simulink model "MLP_networks"  (Simulink 7.7)
settings: Solver=ode45  StartTime=0.0  StopTime=10.0  RelTol=1e-3
libraries: neural x1629
(part 25 of 39)

== system MLP_networks/net_col_e_f_4_5/Layer 2/LW{2,1} ==
  "ad{2,1}" : Inport  PortDimensions=20
      mask Display: e = 0.06;c1 = [120 230 180]/255;c2 = ([120 230 180]+0)/(256+128);c3 = ([120 230 180]+128)/(256+128);patch([0 1 1 0],[0 0 1 1],c1);patch([0 1 1 1-e 1-e 0+e],[0 0 1 1-e 0+e 0+e],c2);patch([0 0 1 1-e 0+e 0+e],[0 1 1 1-e 1-e 0+e],c3);plot([0 1 1 0 0],[0 0 1 1 0]);
  "IW{2,1}(1,:)'" : Constant  Value=[-0.45151548886161508;0.25536682711089687;-0.34681685037556653;-0.34392706874455214;-0.027803182510490278;0.41746512687912851;0.55437397851143355;0.083610404804986299;-0.25747534404557321;-0.31935504733540621;-0.59689163525306344;-0.045683988316651554;-0.43964163854361554;0.11284189827815641;-0.64222573757867818;-0.35635141759648353;0.12263688035408589;-0.58273881801377925;-0.46555293587298402;-0.0080108450108429229]
      mask Display: e = 0.06;c1 = [120 150 230]/255;c2 = ([120 150 230]+0)/383;c3 = ([120 150 230]+128)/383;patch([0 1 1 0],[0 0 1 1],c1);patch([0 1 1 1-e 1-e 0+e],[0 0 1 1-e 0+e 0+e],c2);patch([0 0 1 1-e 0+e 0+e],[0 1 1 1-e 1-e 0+e],c3);plot([0 1 1 0 0],[0 0 1 1 0]);disp('weights');
  "IW{2,1}(10,:)'" : Constant  Value=[0.41523421292602436;-0.079325917445633137;0.60054028682480187;0.54825507956649056;0.042245915117327067;-0.22239028106970385;-0.15170393677920968;-0.28769964161831629;-0.66009683615917791;0.48814562672504147;0.04655942021694514;0.68149765275244589;-0.062084447563797093;-0.47323297326885766;0.22267393118045514;-0.3678342526120863;-0.22194063098682851;0.37035750995645711;0.12347763221984454;-0.31522257591675068]
      mask Display: e = 0.06;c1 = [120 150 230]/255;c2 = ([120 150 230]+0)/383;c3 = ([120 150 230]+128)/383;patch([0 1 1 0],[0 0 1 1],c1);patch([0 1 1 1-e 1-e 0+e],[0 0 1 1-e 0+e 0+e],c2);patch([0 0 1 1-e 0+e 0+e],[0 1 1 1-e 1-e 0+e],c3);plot([0 1 1 0 0],[0 0 1 1 0]);disp('weights');
  "IW{2,1}(11,:)'" : Constant  Value=[0.22051107884975904;0.04667985599907265;-0.42900276186151998;-0.61671126003943155;-0.42621721318611683;-0.18489691728747051;-0.13777397473069228;-0.037474895097715587;0.51799599312536593;-0.084083188529973152;-0.64644464204408958;-0.01135044235336753;-0.070911414979821383;-0.17601825270858257;0.61930700333124977;-0.082126080553112879;0.63071072678260498;0.16527980798998046;0.56344172772425338;0.37422462011786845]
      mask Display: e = 0.06;c1 = [120 150 230]/255;c2 = ([120 150 230]+0)/383;c3 = ([120 150 230]+128)/383;patch([0 1 1 0],[0 0 1 1],c1);patch([0 1 1 1-e 1-e 0+e],[0 0 1 1-e 0+e 0+e],c2);patch([0 0 1 1-e 0+e 0+e],[0 1 1 1-e 1-e 0+e],c3);plot([0 1 1 0 0],[0 0 1 1 0]);disp('weights');
  "IW{2,1}(12,:)'" : Constant  Value=[-0.084493713905112233;0.48678115841687936;0.45142563808834973;-0.36811298581343271;-0.40924916828354552;0.17807058636038001;-0.46456329081936826;0.42281416037711955;0.20377516377164831;0.47843783198352607;-0.26407473415439514;-0.10465597364986522;-0.47919068721275565;0.31496744878274513;0.20713329388106066;0.49180314424343141;0.57605572335121114;-0.22625235422828688;0.46448345523528134;0.27110377760943549]
      mask Display: e = 0.06;c1 = [120 150 230]/255;c2 = ([120 150 230]+0)/383;c3 = ([120 150 230]+128)/383;patch([0 1 1 0],[0 0 1 1],c1);patch([0 1 1 1-e 1-e 0+e],[0 0 1 1-e 0+e 0+e],c2);patch([0 0 1 1-e 0+e 0+e],[0 1 1 1-e 1-e 0+e],c3);plot([0 1 1 0 0],[0 0 1 1 0]);disp('weights');
  "IW{2,1}(13,:)'" : Constant  Value=[-0.30149359766207418;-0.45992478689272992;0.37870307637329009;0.33785088301701416;0.29211040783918429;0.418882893877153;0.52364539021317746;0.22698130724798568;0.41621078446985132;0.32359159164504292;-0.37444769328437505;-0.41424018215945352;0.45640798227554841;0.47255964818598079;0.063960542335897014;-0.33017321165220542;0.25384780898493198;-0.47685133154288806;0.15216466743509105;-0.52149157749906128]
      mask Display: e = 0.06;c1 = [120 150 230]/255;c2 = ([120 150 230]+0)/383;c3 = ([120 150 230]+128)/383;patch([0 1 1 0],[0 0 1 1],c1);patch([0 1 1 1-e 1-e 0+e],[0 0 1 1-e 0+e 0+e],c2);patch([0 0 1 1-e 0+e 0+e],[0 1 1 1-e 1-e 0+e],c3);plot([0 1 1 0 0],[0 0 1 1 0]);disp('weights');
  "IW{2,1}(14,:)'" : Constant  Value=[-0.28930249915012268;-0.44091010774765055;0.27168073044539698;0.49942675426286448;0.20512264087672194;-0.37602605346876733;-0.13189155517247578;-0.23130337724636571;0.094450964076811791;-0.16998091204382224;0.16016055355889927;-0.60759126781458894;0.43104902085232288;-0.56965892606835733;0.17809072069355344;0.28659787509126711;-0.4614072071044088;0.34603812505852033;0.46450688890271252;0.62315023418671689]
      mask Display: e = 0.06;c1 = [120 150 230]/255;c2 = ([120 150 230]+0)/383;c3 = ([120 150 230]+128)/383;patch([0 1 1 0],[0 0 1 1],c1);patch([0 1 1 1-e 1-e 0+e],[0 0 1 1-e 0+e 0+e],c2);patch([0 0 1 1-e 0+e 0+e],[0 1 1 1-e 1-e 0+e],c3);plot([0 1 1 0 0],[0 0 1 1 0]);disp('weights');
  "IW{2,1}(15,:)'" : Constant  Value=[0.15751683268771688;0.4192261852453415;-0.016011679153426196;0.41859753641114317;0.25793731142113935;0.18105600414691669;-0.053963693799016686;-0.56399142195908658;0.28049437874349148;-0.35138609966460516;0.27311840894612877;-0.17274187268768235;-0.23510480251311197;0.61360552858247386;0.73129244534754589;-0.70291713895824193;0.46749838984635617;-0.20341619662205515;0.021850222878550853;-0.12862670708565105]
      mask Display: e = 0.06;c1 = [120 150 230]/255;c2 = ([120 150 230]+0)/383;c3 = ([120 150 230]+128)/383;patch([0 1 1 0],[0 0 1 1],c1);patch([0 1 1 1-e 1-e 0+e],[0 0 1 1-e 0+e 0+e],c2);patch([0 0 1 1-e 0+e 0+e],[0 1 1 1-e 1-e 0+e],c3);plot([0 1 1 0 0],[0 0 1 1 0]);disp('weights');
  "IW{2,1}(16,:)'" : Constant  Value=[-0.27657012366938966;0.15371322358443629;-0.55363356208853609;0.36378906637276537;0.52464494926328686;0.28784110928429885;0.46469559105081931;0.15025065447007821;-0.33039322751314137;-0.06464765041817773;0.20119553589259553;0.133449729104959;0.45132776068432545;0.34991929216206841;-0.40133073823107779;-0.39379744327608268;0.53901406218322345;-0.45996647999988743;-0.4115733283149775;-0.50627799265694229]
      mask Display: e = 0.06;c1 = [120 150 230]/255;c2 = ([120 150 230]+0)/383;c3 = ([120 150 230]+128)/383;patch([0 1 1 0],[0 0 1 1],c1);patch([0 1 1 1-e 1-e 0+e],[0 0 1 1-e 0+e 0+e],c2);patch([0 0 1 1-e 0+e 0+e],[0 1 1 1-e 1-e 0+e],c3);plot([0 1 1 0 0],[0 0 1 1 0]);disp('weights');
  "IW{2,1}(17,:)'" : Constant  Value=[-0.29644152955930081;-0.4308597944950418;-0.54634565930104229;0.58330284826123979;-0.10928909899825232;0.56925501441853865;0.57554506008322792;0.53497171762174578;0.55505559616470479;-0.1148742286263794;-0.53564900218664824;0.044535446781484522;0.20798460923717371;0.29893088797223188;-0.21469482723072089;0.19037112584674373;-0.11652538868178051;0.13763581536126696;0.31150300464310915;-0.094213883008351984]
      mask Display: e = 0.06;c1 = [120 150 230]/255;c2 = ([120 150 230]+0)/383;c3 = ([120 150 230]+128)/383;patch([0 1 1 0],[0 0 1 1],c1);patch([0 1 1 1-e 1-e 0+e],[0 0 1 1-e 0+e 0+e],c2);patch([0 0 1 1-e 0+e 0+e],[0 1 1 1-e 1-e 0+e],c3);plot([0 1 1 0 0],[0 0 1 1 0]);disp('weights');
  "IW{2,1}(18,:)'" : Constant  Value=[0.35417996583849992;0.15868067448218406;-0.35585371797525295;-0.21707074271476465;-0.30874927399822116;0.28469132401145908;0.35472209819061928;0.3415908850634099;-0.55469444381337141;0.35094451772152646;0.70640754781705073;-0.75008386250934855;-0.4794943931696436;-0.21128936679171628;-0.12072435755185078;0.12920961420023977;-0.49022617267297025;-0.38439863878407654;0.21885884977322467;-0.16430755827177285]
      mask Display: e = 0.06;c1 = [120 150 230]/255;c2 = ([120 150 230]+0)/383;c3 = ([120 150 230]+128)/383;patch([0 1 1 0],[0 0 1 1],c1);patch([0 1 1 1-e 1-e 0+e],[0 0 1 1-e 0+e 0+e],c2);patch([0 0 1 1-e 0+e 0+e],[0 1 1 1-e 1-e 0+e],c3);plot([0 1 1 0 0],[0 0 1 1 0]);disp('weights');
  "IW{2,1}(19,:)'" : Constant  Value=[-0.27337498067941102;-0.56335228384022429;-0.053155904668951752;-0.34417360501701988;-0.43978832790699596;-0.5760611884699075;-0.022993975155131994;0.51733797376312773;-0.59073422965442535;-0.32599506194253752;0.39691334336237133;0.59730593053673864;0.51579578103074142;0.18622803089423495;0.22952335035122878;0.28644120269709844;-0.022213765514939521;0.70000625526608418;-0.18510048875217902;0.13283311097415057]
      mask Display: e = 0.06;c1 = [120 150 230]/255;c2 = ([120 150 230]+0)/383;c3 = ([120 150 230]+128)/383;patch([0 1 1 0],[0 0 1 1],c1);patch([0 1 1 1-e 1-e 0+e],[0 0 1 1-e 0+e 0+e],c2);patch([0 0 1 1-e 0+e 0+e],[0 1 1 1-e 1-e 0+e],c3);plot([0 1 1 0 0],[0 0 1 1 0]);disp('weights');
  "IW{2,1}(2,:)'" : Constant  Value=[0.28437748977449745;0.25833400523463534;-0.037021315231732362;-0.68497084905838668;0.41852802820217722;-0.57834088769097802;0.56203903722750315;-0.21187070828271204;-0.10478414525478082;0.57659603478192067;-0.7418424500897558;-0.39611970693280452;0.069829662330228442;-0.15617944332060318;0.25357993180904392;-0.065271231016431744;0.31908541214869918;-0.060339638688504026;0.081335933949920322;-0.37526662583148929]
      mask Display: e = 0.06;c1 = [120 150 230]/255;c2 = ([120 150 230]+0)/383;c3 = ([120 150 230]+128)/383;patch([0 1 1 0],[0 0 1 1],c1);patch([0 1 1 1-e 1-e 0+e],[0 0 1 1-e 0+e 0+e],c2);patch([0 0 1 1-e 0+e 0+e],[0 1 1 1-e 1-e 0+e],c3);plot([0 1 1 0 0],[0 0 1 1 0]);disp('weights');
  "IW{2,1}(20,:)'" : Constant  Value=[-0.64409750347750527;0.34646163018063469;-0.58798361872778426;0.0085129432317137699;-0.45090915364862233;-0.30265599114041347;0.0077096397280898114;0.26412412391892426;0.086341121032416118;-0.30548428858564097;0.3660050363044266;-0.62694176855105233;-0.48252047203090886;-0.52245941640535487;0.38730598212166212;-0.064531981023332644;0.17425424198955766;0.53562209298160957;-0.061191832450063051;0.043829994940977078]
      mask Display: e = 0.06;c1 = [120 150 230]/255;c2 = ([120 150 230]+0)/383;c3 = ([120 150 230]+128)/383;patch([0 1 1 0],[0 0 1 1],c1);patch([0 1 1 1-e 1-e 0+e],[0 0 1 1-e 0+e 0+e],c2);patch([0 0 1 1-e 0+e 0+e],[0 1 1 1-e 1-e 0+e],c3);plot([0 1 1 0 0],[0 0 1 1 0]);disp('weights');
  "IW{2,1}(21,:)'" : Constant  Value=[-0.080332203363595853;0.37070858702897092;0.23410866955263651;0.26082762551266808;-0.46717907369368694;-0.50512936006521436;0.45092995928204604;-0.51896037678346807;-0.56100829375195771;0.21814326179802759;0.040103435817852924;0.17387153933872629;-0.13079318849718519;0.61280554963107803;-0.31277142209582232;-0.39206937616288345;0.37537171334969721;-0.075970000529032425;0.41224430106766913;0.52254642336293189]
      mask Display: e = 0.06;c1 = [120 150 230]/255;c2 = ([120 150 230]+0)/383;c3 = ([120 150 230]+128)/383;patch([0 1 1 0],[0 0 1 1],c1);patch([0 1 1 1-e 1-e 0+e],[0 0 1 1-e 0+e 0+e],c2);patch([0 0 1 1-e 0+e 0+e],[0 1 1 1-e 1-e 0+e],c3);plot([0 1 1 0 0],[0 0 1 1 0]);disp('weights');
  "IW{2,1}(22,:)'" : Constant  Value=[-0.42704336720470931;-0.30041882948731219;0.3956809292562421;-0.16971732971577322;0.076497757409530881;-0.47929628792147649;-0.24193017744364609;-0.247136213895218;0.07517234050153429;0.10672754370040455;-0.36319238605476445;0.97284045806936903;0.048026106182699771;0.42305021233232182;-0.46384915148240169;-0.41910492272950939;-0.64315109777288715;-0.4816034710376344;-0.1382623929613658;0.43671260004494816]
      mask Display: e = 0.06;c1 = [120 150 230]/255;c2 = ([120 150 230]+0)/383;c3 = ([120 150 230]+128)/383;patch([0 1 1 0],[0 0 1 1],c1);patch([0 1 1 1-e 1-e 0+e],[0 0 1 1-e 0+e 0+e],c2);patch([0 0 1 1-e 0+e 0+e],[0 1 1 1-e 1-e 0+e],c3);plot([0 1 1 0 0],[0 0 1 1 0]);disp('weights');
  "IW{2,1}(23,:)'" : Constant  Value=[0.43259582298602201;0.085300864815750416;-0.066611187728102428;-0.46644934301614377;0.56800532870993614;-0.16825181379550211;0.065952412563121496;0.067656163269610964;0.46000807496535551;-0.54532641650351965;0.48758798102992756;0.0079347445270282254;-0.24701594877729452;0.40742904315943818;0.5647408817287688;-0.15873910115094836;-0.18642398510228386;0.40592279947701382;0.59479591210183047;-0.43874366904786444]
      mask Display: e = 0.06;c1 = [120 150 230]/255;c2 = ([120 150 230]+0)/383;c3 = ([120 150 230]+128)/383;patch([0 1 1 0],[0 0 1 1],c1);patch([0 1 1 1-e 1-e 0+e],[0 0 1 1-e 0+e 0+e],c2);patch([0 0 1 1-e 0+e 0+e],[0 1 1 1-e 1-e 0+e],c3);plot([0 1 1 0 0],[0 0 1 1 0]);disp('weights');
  "IW{2,1}(24,:)'" : Constant  Value=[0.19016036357024163;0.57929888615100023;-0.14047319816385875;0.038995668949996558;-0.44390268551296003;0.30519117481283614;-0.34432327516636352;-0.37456076679867462;0.54440803834519624;-0.019815912098819614;0.63106674401813323;0.37836063975903239;0.065211801093335867;0.19335193979332421;0.63042804000337915;0.28047911862511621;0.5187382647019726;0.028624368762329815;-0.43731282398140586;-0.26967529965222736]
      mask Display: e = 0.06;c1 = [120 150 230]/255;c2 = ([120 150 230]+0)/383;c3 = ([120 150 230]+128)/383;patch([0 1 1 0],[0 0 1 1],c1);patch([0 1 1 1-e 1-e 0+e],[0 0 1 1-e 0+e 0+e],c2);patch([0 0 1 1-e 0+e 0+e],[0 1 1 1-e 1-e 0+e],c3);plot([0 1 1 0 0],[0 0 1 1 0]);disp('weights');
  "IW{2,1}(25,:)'" : Constant  Value=[-0.50936038839145192;-0.19277928465516786;0.098729651458946244;0.53123727125983733;-0.58577391142315827;0.067452152417218442;-0.60444589710104868;0.035797191391837291;0.15815085104115664;0.42816638333026946;-0.54946945388590596;0.041608575715513151;-0.18465440432688701;0.222307296844788;-0.52045372767096176;-0.52995581953262583;0.26174237394350625;0.38065149951346616;-0.16035256651239119;-0.43015951076477787]
      mask Display: e = 0.06;c1 = [120 150 230]/255;c2 = ([120 150 230]+0)/383;c3 = ([120 150 230]+128)/383;patch([0 1 1 0],[0 0 1 1],c1);patch([0 1 1 1-e 1-e 0+e],[0 0 1 1-e 0+e 0+e],c2);patch([0 0 1 1-e 0+e 0+e],[0 1 1 1-e 1-e 0+e],c3);plot([0 1 1 0 0],[0 0 1 1 0]);disp('weights');
  "IW{2,1}(26,:)'" : Constant  Value=[0.49161235461354219;0.13938404534825224;0.19689113128497887;-0.57832411689609775;0.20308506261153095;0.62481272330751148;-0.1163707285325393;-0.37825325200630266;0.48294919143002357;0.014653694283724624;0.22084013857339119;-0.30477867491497423;-0.51827876473227408;-0.024621345595192568;0.66148074875242446;0.075740436850787865;0.1204109369260714;-0.63548975553075482;0.38742754064669516;-0.14709552917403249]
      mask Display: e = 0.06;c1 = [120 150 230]/255;c2 = ([120 150 230]+0)/383;c3 = ([120 150 230]+128)/383;patch([0 1 1 0],[0 0 1 1],c1);patch([0 1 1 1-e 1-e 0+e],[0 0 1 1-e 0+e 0+e],c2);patch([0 0 1 1-e 0+e 0+e],[0 1 1 1-e 1-e 0+e],c3);plot([0 1 1 0 0],[0 0 1 1 0]);disp('weights');
  "IW{2,1}(27,:)'" : Constant  Value=[0.019138504382321172;0.28381222077012969;-0.49604976359267183;-0.28449537899504079;-0.41733198679167754;0.092655965391060455;0.18812170443162871;0.19957812537122963;0.36569212890338643;0.46823789772659924;-0.076708279733774296;-0.22357230424429589;-0.64292437440370276;0.46401462443333891;0.44379639158890594;0.41954559118593693;0.55890697457605876;0.11240640528838934;-0.30265224534970631;-0.5528095628665205]
      mask Display: e = 0.06;c1 = [120 150 230]/255;c2 = ([120 150 230]+0)/383;c3 = ([120 150 230]+128)/383;patch([0 1 1 0],[0 0 1 1],c1);patch([0 1 1 1-e 1-e 0+e],[0 0 1 1-e 0+e 0+e],c2);patch([0 0 1 1-e 0+e 0+e],[0 1 1 1-e 1-e 0+e],c3);plot([0 1 1 0 0],[0 0 1 1 0]);disp('weights');
  "IW{2,1}(28,:)'" : Constant  Value=[-0.46483245257272948;0.42495318046244368;0.43385144514194263;0.5795355145128539;-0.31719114707076268;-0.025928385016244816;0.55529060554396115;0.48985316366965981;0.19365713029830708;-0.27863440317519872;0.17818812619051516;-0.13994906307191879;-0.35004184669492061;0.21193774460530071;0.2014304792059381;-0.58966967725916897;-0.28919171380182246;-0.17419785067078189;-0.55783273516298526;0.34599451625435185]
      mask Display: e = 0.06;c1 = [120 150 230]/255;c2 = ([120 150 230]+0)/383;c3 = ([120 150 230]+128)/383;patch([0 1 1 0],[0 0 1 1],c1);patch([0 1 1 1-e 1-e 0+e],[0 0 1 1-e 0+e 0+e],c2);patch([0 0 1 1-e 0+e 0+e],[0 1 1 1-e 1-e 0+e],c3);plot([0 1 1 0 0],[0 0 1 1 0]);disp('weights');
  "IW{2,1}(29,:)'" : Constant  Value=[0.077132854850568561;0.42893800153588429;0.30188800684931705;-0.51335827552667535;-0.52741869534436991;0.52774124253488452;0.049069872655798388;-0.38359828687075909;0.28178370735123903;0.50235556529196024;0.082418447614783855;0.29838163528191525;0.24944756358228873;0.3987895979494982;-0.24319839906119098;-0.45168734003488942;0.30889583270709497;0.43599021698063084;0.37267528447680792;0.51943087246993669]
      mask Display: e = 0.06;c1 = [120 150 230]/255;c2 = ([120 150 230]+0)/383;c3 = ([120 150 230]+128)/383;patch([0 1 1 0],[0 0 1 1],c1);patch([0 1 1 1-e 1-e 0+e],[0 0 1 1-e 0+e 0+e],c2);patch([0 0 1 1-e 0+e 0+e],[0 1 1 1-e 1-e 0+e],c3);plot([0 1 1 0 0],[0 0 1 1 0]);disp('weights');
  "IW{2,1}(3,:)'" : Constant  Value=[0.11171449310470105;0.013839760390359371;-0.390987297822663;-0.37451899143526957;0.27821065465227218;0.80500660766775156;-0.1209127890345735;0.79070972594755584;-0.18340993997233074;-0.21705292666272946;-0.53957667626884309;0.18883293917454819;-0.30669291691506567;-0.28385551728869829;0.11930455933169529;0.055609117887027694;-0.30578055956435019;0.42271963186133144;-0.35772760583274493;-0.40253190007293055]
      mask Display: e = 0.06;c1 = [120 150 230]/255;c2 = ([120 150 230]+0)/383;c3 = ([120 150 230]+128)/383;patch([0 1 1 0],[0 0 1 1],c1);patch([0 1 1 1-e 1-e 0+e],[0 0 1 1-e 0+e 0+e],c2);patch([0 0 1 1-e 0+e 0+e],[0 1 1 1-e 1-e 0+e],c3);plot([0 1 1 0 0],[0 0 1 1 0]);disp('weights');
  "IW{2,1}(30,:)'" : Constant  Value=[-0.27448265936562655;0.48183133717029614;-0.58858464409181621;0.24886661672157895;-0.52221065400431421;-0.34236118922421704;-0.3408382343466031;0.23658999842474371;0.35377417274944833;0.026388880195584934;-0.4307323462072587;-0.33755650890347294;0.4259208024209003;-0.57404298672102705;0.26729813944772945;-0.48157672602734103;-0.13695964470358912;0.45610479971151474;0.20261152537475213;0.25030727672508368]
      mask Display: e = 0.06;c1 = [120 150 230]/255;c2 = ([120 150 230]+0)/383;c3 = ([120 150 230]+128)/383;patch([0 1 1 0],[0 0 1 1],c1);patch([0 1 1 1-e 1-e 0+e],[0 0 1 1-e 0+e 0+e],c2);patch([0 0 1 1-e 0+e 0+e],[0 1 1 1-e 1-e 0+e],c3);plot([0 1 1 0 0],[0 0 1 1 0]);disp('weights');
  "IW{2,1}(31,:)'" : Constant  Value=[0.5067260022538862;0.34486542778986001;0.29856817351021231;-0.38908971230658118;-0.13793422797340091;-0.31713470092343848;0.15506496026787739;0.23017987565327366;0.36626953658368766;0.47207146604137901;0.26942496621336171;-0.282750578748659;0.32563569504990153;0.1858688848206323;-0.55097539615872759;-0.53486836065354537;0.52026592924190806;-0.41135207441526295;0.53288672107383428;-0.222159875686782]
      mask Display: e = 0.06;c1 = [120 150 230]/255;c2 = ([120 150 230]+0)/383;c3 = ([120 150 230]+128)/383;patch([0 1 1 0],[0 0 1 1],c1);patch([0 1 1 1-e 1-e 0+e],[0 0 1 1-e 0+e 0+e],c2);patch([0 0 1 1-e 0+e 0+e],[0 1 1 1-e 1-e 0+e],c3);plot([0 1 1 0 0],[0 0 1 1 0]);disp('weights');
  "IW{2,1}(32,:)'" : Constant  Value=[-0.19774638934387787;0.69239772756946993;-0.16053889494318915;0.12270358184034273;0.55864383601039425;-0.13008444484939641;0.0083575255006178052;-0.11901874580309373;0.25219449399893262;0.38694465463846411;-0.24672245982359009;0.63818952088119618;0.43783965085744647;0.6829007110946872;0.3670299235507426;-0.33714675816369227;-0.32551091534694987;-0.38691894243056174;-0.43749924089161024;-0.20657291049284418]
      mask Display: e = 0.06;c1 = [120 150 230]/255;c2 = ([120 150 230]+0)/383;c3 = ([120 150 230]+128)/383;patch([0 1 1 0],[0 0 1 1],c1);patch([0 1 1 1-e 1-e 0+e],[0 0 1 1-e 0+e 0+e],c2);patch([0 0 1 1-e 0+e 0+e],[0 1 1 1-e 1-e 0+e],c3);plot([0 1 1 0 0],[0 0 1 1 0]);disp('weights');
  "IW{2,1}(33,:)'" : Constant  Value=[-0.61696116594174;0.51363147456266445;-0.12110893903203764;0.46378638100339509;0.54459998818448851;-0.39400047540247657;-0.40511298968487491;-0.26105030383598077;0.086325847376248099;0.355914796613924;-0.20852108310619924;0.16009958329489335;0.49261679115334822;-0.46447915323937222;0.54451936706386195;-0.28668469325114354;0.050863140194635476;0.3209871472325399;0.11158709955998268;0.35784649388757489]
      mask Display: e = 0.06;c1 = [120 150 230]/255;c2 = ([120 150 230]+0)/383;c3 = ([120 150 230]+128)/383;patch([0 1 1 0],[0 0 1 1],c1);patch([0 1 1 1-e 1-e 0+e],[0 0 1 1-e 0+e 0+e],c2);patch([0 0 1 1-e 0+e 0+e],[0 1 1 1-e 1-e 0+e],c3);plot([0 1 1 0 0],[0 0 1 1 0]);disp('weights');
  "IW{2,1}(34,:)'" : Constant  Value=[0.47425672824242299;-0.26621996182255181;-0.19360955281478065;0.3808149152185723;-0.42208611840162868;-0.42817899001556731;-0.40716715728582364;-0.45028745115232438;-0.00014657021574923215;-0.015581253560115967;-0.71378535547139199;0.5260929231347109;-0.25805419894864734;-0.48780376663300251;-0.023880074529700028;0.53628126352106664;0.43454983765857075;-0.0082252387926057755;-0.47714880694570749;-0.40076177909238786]
      mask Display: e = 0.06;c1 = [120 150 230]/255;c2 = ([120 150 230]+0)/383;c3 = ([120 150 230]+128)/383;patch([0 1 1 0],[0 0 1 1],c1);patch([0 1 1 1-e 1-e 0+e],[0 0 1 1-e 0+e 0+e],c2);patch([0 0 1 1-e 0+e 0+e],[0 1 1 1-e 1-e 0+e],c3);plot([0 1 1 0 0],[0 0 1 1 0]);disp('weights');
  "IW{2,1}(35,:)'" : Constant  Value=[-0.53454678185013393;0.5944929064215233;-0.29406982189084663;-0.18970120928103562;0.0092461234286018885;-0.38680589954760142;-0.49700772169234891;-0.05201111652998644;0.053517501299979786;0.25409070724540467;0.1497662875744038;-0.55342103145804367;-0.65409003325717363;0.22928854944584603;0.25060416025194432;-0.18428962968015328;0.27399520345642753;0.45541366346054407;0.53432417632271456;-0.36802000030700294]
      mask Display: e = 0.06;c1 = [120 150 230]/255;c2 = ([120 150 230]+0)/383;c3 = ([120 150 230]+128)/383;patch([0 1 1 0],[0 0 1 1],c1);patch([0 1 1 1-e 1-e 0+e],[0 0 1 1-e 0+e 0+e],c2);patch([0 0 1 1-e 0+e 0+e],[0 1 1 1-e 1-e 0+e],c3);plot([0 1 1 0 0],[0 0 1 1 0]);disp('weights');
  "IW{2,1}(36,:)'" : Constant  Value=[-0.13222099654614625;-0.57903462850803233;-0.089984780231621569;0.20241667736304428;-0.5672202582908189;-0.34762806709331351;0.09972790031357566;-0.32317144892521033;-0.7788395685290288;0.48107159653025794;-0.24977990819171875;0.020065834811667235;-0.45166547353796993;-0.40304756316969598;0.11503747528317694;0.20101407326350687;-0.40293709810902489;0.46277598013813087;0.37455439588983586;-0.18908737960287403]
      mask Display: e = 0.06;c1 = [120 150 230]/255;c2 = ([120 150 230]+0)/383;c3 = ([120 150 230]+128)/383;patch([0 1 1 0],[0 0 1 1],c1);patch([0 1 1 1-e 1-e 0+e],[0 0 1 1-e 0+e 0+e],c2);patch([0 0 1 1-e 0+e 0+e],[0 1 1 1-e 1-e 0+e],c3);plot([0 1 1 0 0],[0 0 1 1 0]);disp('weights');
  "IW{2,1}(37,:)'" : Constant  Value=[-0.27683574345437378;0.28651029496602448;-0.76362458797023769;-0.20670188616307122;-0.13598676665432433;-0.15183317133947841;0.32848298757552674;0.19528873687846326;-0.32014017404590422;0.36325395153141105;-0.45010979847029092;-0.3710875612250284;1.1204161563103043;0.31427927634464092;0.485504145989265;0.10623212474618046;-0.0092987531657891444;-0.16878284444660632;-0.043993975605504318;-3.2331162802376865e-005]
      mask Display: e = 0.06;c1 = [120 150 230]/255;c2 = ([120 150 230]+0)/383;c3 = ([120 150 230]+128)/383;patch([0 1 1 0],[0 0 1 1],c1);patch([0 1 1 1-e 1-e 0+e],[0 0 1 1-e 0+e 0+e],c2);patch([0 0 1 1-e 0+e 0+e],[0 1 1 1-e 1-e 0+e],c3);plot([0 1 1 0 0],[0 0 1 1 0]);disp('weights');
  "IW{2,1}(38,:)'" : Constant  Value=[-0.039428993484827361;-0.67357952085438544;-0.19855618491303709;0.087005648169222308;0.23112843287667156;-0.51384293801628922;0.18642013757683726;-0.67942216427967606;-0.06689573512727133;-0.73792447956453777;0.39855736950186899;-0.10783028158674163;0.46390231602689197;-0.32788755358261173;-0.30593148866216274;0.33661832485509785;-0.2211955511742825;0.5160706097056722;-0.42579594206007648;-0.35694386995218569]
      mask Display: e = 0.06;c1 = [120 150 230]/255;c2 = ([120 150 230]+0)/383;c3 = ([120 150 230]+128)/383;patch([0 1 1 0],[0 0 1 1],c1);patch([0 1 1 1-e 1-e 0+e],[0 0 1 1-e 0+e 0+e],c2);patch([0 0 1 1-e 0+e 0+e],[0 1 1 1-e 1-e 0+e],c3);plot([0 1 1 0 0],[0 0 1 1 0]);disp('weights');
  "IW{2,1}(39,:)'" : Constant  Value=[-0.45049336636226006;-0.5367493291383304;0.044990087776488094;0.046641281528807109;-0.26311779182964579;-0.13334052078642611;0.24308207470765314;-0.46246542901194493;0.35792749421697523;-0.37475390858823687;0.25948086458092084;0.41300986517206717;0.10476593102880249;-0.062529324070357703;-0.46771588576581136;0.48874872608141096;0.47021691779148278;0.53802282640291743;0.39473298428946885;-0.53412370660207198]
      mask Display: e = 0.06;c1 = [120 150 230]/255;c2 = ([120 150 230]+0)/383;c3 = ([120 150 230]+128)/383;patch([0 1 1 0],[0 0 1 1],c1);patch([0 1 1 1-e 1-e 0+e],[0 0 1 1-e 0+e 0+e],c2);patch([0 0 1 1-e 0+e 0+e],[0 1 1 1-e 1-e 0+e],c3);plot([0 1 1 0 0],[0 0 1 1 0]);disp('weights');
  "IW{2,1}(4,:)'" : Constant  Value=[0.39966796877481714;-0.54988696757707067;-0.50310783022284333;-0.53396216474072389;-0.13060412083919562;0.38740640503267015;-0.10702469844270321;-0.4368512887685031;-0.33272470752672378;-0.088458445995512031;-0.52576477178629211;0.22804645753654459;-0.14694076834914857;0.19440604023168517;0.50077340626474054;0.094203143834088454;0.27210558696816622;-0.47601530112021379;0.43724066090794639;-0.51468730506518257]
      mask Display: e = 0.06;c1 = [120 150 230]/255;c2 = ([120 150 230]+0)/383;c3 = ([120 150 230]+128)/383;patch([0 1 1 0],[0 0 1 1],c1);patch([0 1 1 1-e 1-e 0+e],[0 0 1 1-e 0+e 0+e],c2);patch([0 0 1 1-e 0+e 0+e],[0 1 1 1-e 1-e 0+e],c3);plot([0 1 1 0 0],[0 0 1 1 0]);disp('weights');
  "IW{2,1}(40,:)'" : Constant  Value=[-0.43173174481697518;-0.2758633627331023;0.37451952027209873;-0.41046370246008684;-0.14801730497225313;-0.045485284202633779;0.01483176915025573;0.47290472959979624;0.67778890112494405;0.46279058806999895;-0.25781862373483844;0.19009458645433641;0.54222060953459317;-0.068301077978920988;-0.13636688976859695;-0.37554959360139578;0.25653429367733799;0.4057619481045156;-0.59132354603894921;0.36722852270131445]
      mask Display: e = 0.06;c1 = [120 150 230]/255;c2 = ([120 150 230]+0)/383;c3 = ([120 150 230]+128)/383;patch([0 1 1 0],[0 0 1 1],c1);patch([0 1 1 1-e 1-e 0+e],[0 0 1 1-e 0+e 0+e],c2);patch([0 0 1 1-e 0+e 0+e],[0 1 1 1-e 1-e 0+e],c3);plot([0 1 1 0 0],[0 0 1 1 0]);disp('weights');
  "IW{2,1}(5,:)'" : Constant  Value=[0.35567997938553658;0.23842379774848552;0.40771837618502871;-0.47517848467483065;-0.39880094653635351;-0.2699151102995116;0.64947151860241248;0.17058543982668881;0.61045906551530416;0.51183445780718451;0.20823147623925553;-0.046829920408593788;0.1002429496352691;0.2671163786867059;-0.21106202525212497;0.24676853660494699;0.16292762114169115;-0.28586590655297628;0.32062689324860527;-0.62685279482333678]
      mask Display: e = 0.06;c1 = [120 150 230]/255;c2 = ([120 150 230]+0)/383;c3 = ([120 150 230]+128)/383;patch([0 1 1 0],[0 0 1 1],c1);patch([0 1 1 1-e 1-e 0+e],[0 0 1 1-e 0+e 0+e],c2);patch([0 0 1 1-e 0+e 0+e],[0 1 1 1-e 1-e 0+e],c3);plot([0 1 1 0 0],[0 0 1 1 0]);disp('weights');
  "IW{2,1}(6,:)'" : Constant  Value=[-0.51401666710099903;-0.43547581342373098;0.42719605870999466;-0.4451997720060068;-0.10961971869687816;0.081892645646542986;0.5021926395196149;0.41449256192859962;0.22631409985886786;0.47425916172821508;-0.33866853951241083;0.48164343503706364;0.20285783262909746;-0.13920836951662985;-0.50717218883583115;-0.52246162415414144;0.4351138430538104;-0.052173128241893275;0.27382438524289671;0.2770924555593357]
      mask Display: e = 0.06;c1 = [120 150 230]/255;c2 = ([120 150 230]+0)/383;c3 = ([120 150 230]+128)/383;patch([0 1 1 0],[0 0 1 1],c1);patch([0 1 1 1-e 1-e 0+e],[0 0 1 1-e 0+e 0+e],c2);patch([0 0 1 1-e 0+e 0+e],[0 1 1 1-e 1-e 0+e],c3);plot([0 1 1 0 0],[0 0 1 1 0]);disp('weights');
  "IW{2,1}(7,:)'" : Constant  Value=[-0.11633538490477187;-0.42482367150278522;-0.62378681713537165;0.18427766671983134;-0.37767144714944778;-0.037002229874999189;0.37870010280345684;0.32641284989145103;-0.6096613176442881;0.66372200870281806;0.65525362365790984;0.06492440817289831;-0.49204612422648897;-0.14220149698358298;-0.0025093214907876585;-0.52131178938332778;-0.16654437992180654;0.56753783412984715;0.67691348041063182;0.10812300560089746]
      mask Display: e = 0.06;c1 = [120 150 230]/255;c2 = ([120 150 230]+0)/383;c3 = ([120 150 230]+128)/383;patch([0 1 1 0],[0 0 1 1],c1);patch([0 1 1 1-e 1-e 0+e],[0 0 1 1-e 0+e 0+e],c2);patch([0 0 1 1-e 0+e 0+e],[0 1 1 1-e 1-e 0+e],c3);plot([0 1 1 0 0],[0 0 1 1 0]);disp('weights');
  "IW{2,1}(8,:)'" : Constant  Value=[-0.28732359644826921;0.15195376571767061;0.53198762414018752;0.23886508208314711;-0.34895777094145775;-0.11485624646185499;0.35502049132573738;0.79726647465073475;0.30438815508461686;-0.46518522620631825;0.079608927566267959;0.28719755551394804;0.693852973485102;0.40990280356490022;0.12943506161235643;0.11386395946826619;-0.23220671310713556;0.42950649715630923;-0.0073788518514367385;0.16868184934485089]
      mask Display: e = 0.06;c1 = [120 150 230]/255;c2 = ([120 150 230]+0)/383;c3 = ([120 150 230]+128)/383;patch([0 1 1 0],[0 0 1 1],c1);patch([0 1 1 1-e 1-e 0+e],[0 0 1 1-e 0+e 0+e],c2);patch([0 0 1 1-e 0+e 0+e],[0 1 1 1-e 1-e 0+e],c3);plot([0 1 1 0 0],[0 0 1 1 0]);disp('weights');
  "IW{2,1}(9,:)'" : Constant  Value=[-0.50929426110369636;0.17011294673194538;0.3821493672992694;-0.27596967718475446;0.33996233357043026;-0.54641049566113109;-0.56434619142233056;-0.0027557008027561903;0.35392034028986136;-0.41643372802953971;0.27530185796870638;0.31711372494573609;-0.20951880276774049;-0.18504102831381208;0.32925051678692269;0.40511078069412798;0.53820174637586471;0.090386319323031386;-0.46766800712541501;0.40465405026203977]
      mask Display: e = 0.06;c1 = [120 150 230]/255;c2 = ([120 150 230]+0)/383;c3 = ([120 150 230]+128)/383;patch([0 1 1 0],[0 0 1 1],c1);patch([0 1 1 1-e 1-e 0+e],[0 0 1 1-e 0+e 0+e],c2);patch([0 0 1 1-e 0+e 0+e],[0 1 1 1-e 1-e 0+e],c3);plot([0 1 1 0 0],[0 0 1 1 0]);disp('weights');
  Mux : Mux  Inputs=40
      mask Display: e = 0.06;c1 = [120 150 230]/255;c2 = ([120 150 230]+0)/383;c3 = ([120 150 230]+128)/383;patch([0 1 1 0],[0 0 1 1],c1);patch([0 1 1 1-e 1-e 0+e],[0 0 1 1-e 0+e 0+e],c2);patch([0 0 1 1-e 0+e 0+e],[0 1 1 1-e 1-e 0+e],c3);plot([0 1 1 0 0],[0 0 1 1 0]);disp('Mux');
  dotprod{1..40} (40 alike) : neural/Weight Functions/dotprod  SystemSampleTime=-1
  "lz{2,1}" : Outport
      mask Display: e = 0.06;c1 = [120 230 180]/255;c2 = ([120 230 180]+0)/(256+128);c3 = ([120 230 180]+128)/(256+128);patch([0 1 1 0],[0 0 1 1],c1);patch([0 1 1 1-e 1-e 0+e],[0 0 1 1-e 0+e 0+e],c2);patch([0 0 1 1-e 0+e 0+e],[0 1 1 1-e 1-e 0+e],c3);plot([0 1 1 0 0],[0 0 1 1 0]);
  wires:
  "IW{2,1}(1,:)'"/1 -> dotprod1/1
  "ad{2,1}"/1 -> dotprod1/2, dotprod2/2, dotprod3/2, dotprod4/2, dotprod5/2, dotprod6/2, dotprod7/2, dotprod8/2, dotprod9/2, dotprod10/2, dotprod11/2, dotprod12/2, dotprod13/2, dotprod14/2, dotprod15/2, dotprod16/2, dotprod17/2, dotprod18/2, dotprod19/2, dotprod20/2, dotprod21/2, dotprod22/2, dotprod23/2, dotprod24/2, dotprod25/2, dotprod26/2, dotprod27/2, dotprod28/2, dotprod29/2, dotprod30/2, dotprod31/2, dotprod32/2, dotprod33/2, dotprod34/2, dotprod35/2, dotprod36/2, dotprod37/2, dotprod38/2, dotprod39/2, dotprod40/2
  dotprod1/1 -> Mux/1
  "IW{2,1}(2,:)'"/1 -> dotprod2/1
  dotprod2/1 -> Mux/2
  "IW{2,1}(3,:)'"/1 -> dotprod3/1
  dotprod3/1 -> Mux/3
  "IW{2,1}(4,:)'"/1 -> dotprod4/1
  dotprod4/1 -> Mux/4
  "IW{2,1}(5,:)'"/1 -> dotprod5/1
  dotprod5/1 -> Mux/5
  "IW{2,1}(6,:)'"/1 -> dotprod6/1
  dotprod6/1 -> Mux/6
  "IW{2,1}(7,:)'"/1 -> dotprod7/1
  dotprod7/1 -> Mux/7
  "IW{2,1}(8,:)'"/1 -> dotprod8/1
  dotprod8/1 -> Mux/8
  "IW{2,1}(9,:)'"/1 -> dotprod9/1
  dotprod9/1 -> Mux/9
  "IW{2,1}(10,:)'"/1 -> dotprod10/1
  dotprod10/1 -> Mux/10
  "IW{2,1}(11,:)'"/1 -> dotprod11/1
  dotprod11/1 -> Mux/11
  "IW{2,1}(12,:)'"/1 -> dotprod12/1
  dotprod12/1 -> Mux/12
  "IW{2,1}(13,:)'"/1 -> dotprod13/1
  dotprod13/1 -> Mux/13
  "IW{2,1}(14,:)'"/1 -> dotprod14/1
  dotprod14/1 -> Mux/14
  "IW{2,1}(15,:)'"/1 -> dotprod15/1
  dotprod15/1 -> Mux/15
  "IW{2,1}(16,:)'"/1 -> dotprod16/1
  dotprod16/1 -> Mux/16
  "IW{2,1}(17,:)'"/1 -> dotprod17/1
  dotprod17/1 -> Mux/17
  "IW{2,1}(18,:)'"/1 -> dotprod18/1
  dotprod18/1 -> Mux/18
  "IW{2,1}(19,:)'"/1 -> dotprod19/1
  dotprod19/1 -> Mux/19
  "IW{2,1}(20,:)'"/1 -> dotprod20/1
  dotprod20/1 -> Mux/20
  "IW{2,1}(21,:)'"/1 -> dotprod21/1
  dotprod21/1 -> Mux/21
  "IW{2,1}(22,:)'"/1 -> dotprod22/1
  dotprod22/1 -> Mux/22
  "IW{2,1}(23,:)'"/1 -> dotprod23/1
  dotprod23/1 -> Mux/23
  "IW{2,1}(24,:)'"/1 -> dotprod24/1
  dotprod24/1 -> Mux/24
  "IW{2,1}(25,:)'"/1 -> dotprod25/1
  dotprod25/1 -> Mux/25
  "IW{2,1}(26,:)'"/1 -> dotprod26/1
  dotprod26/1 -> Mux/26
  "IW{2,1}(27,:)'"/1 -> dotprod27/1
  dotprod27/1 -> Mux/27
  "IW{2,1}(28,:)'"/1 -> dotprod28/1
  dotprod28/1 -> Mux/28
  "IW{2,1}(29,:)'"/1 -> dotprod29/1
  dotprod29/1 -> Mux/29
  "IW{2,1}(30,:)'"/1 -> dotprod30/1
  dotprod30/1 -> Mux/30
  "IW{2,1}(31,:)'"/1 -> dotprod31/1
  dotprod31/1 -> Mux/31
  "IW{2,1}(32,:)'"/1 -> dotprod32/1
  dotprod32/1 -> Mux/32
  "IW{2,1}(33,:)'"/1 -> dotprod33/1
  dotprod33/1 -> Mux/33
  "IW{2,1}(34,:)'"/1 -> dotprod34/1
  dotprod34/1 -> Mux/34
  "IW{2,1}(35,:)'"/1 -> dotprod35/1
  dotprod35/1 -> Mux/35
  "IW{2,1}(36,:)'"/1 -> dotprod36/1
  dotprod36/1 -> Mux/36
  "IW{2,1}(37,:)'"/1 -> dotprod37/1
  dotprod37/1 -> Mux/37
  "IW{2,1}(38,:)'"/1 -> dotprod38/1
  dotprod38/1 -> Mux/38
  "IW{2,1}(39,:)'"/1 -> dotprod39/1
  dotprod39/1 -> Mux/39
  "IW{2,1}(40,:)'"/1 -> dotprod40/1
  dotprod40/1 -> Mux/40
  Mux/1 -> "lz{2,1}"/1

== system MLP_networks/net_col_e_f_4_5/Layer 3/Delays 1 ==
  "p{3}" : Inport  PortDimensions=40
      mask Display: e = 0.06;c1 = [120 230 180]/255;c2 = ([120 230 180]+0)/(256+128);c3 = ([120 230 180]+128)/(256+128);patch([0 1 1 0],[0 0 1 1],c1);patch([0 1 1 1-e 1-e 0+e],[0 0 1 1-e 0+e 0+e],c2);patch([0 0 1 1-e 0+e 0+e],[0 1 1 1-e 1-e 0+e],c3);plot([0 1 1 0 0],[0 0 1 1 0]);
  mux : Mux  Inputs=1
      mask Display: e = 0.06;c1 = [120 150 230]/255;c2 = ([120 150 230]+0)/383;c3 = ([120 150 230]+128)/383;patch([0 1 1 0],[0 0 1 1],c1);patch([0 1 1 1-e 1-e 0+e],[0 0 1 1-e 0+e 0+e],c2);patch([0 0 1 1-e 0+e 0+e],[0 1 1 1-e 1-e 0+e],c3);plot([0 1 1 0 0],[0 0 1 1 0]);disp('Mux')
  "pd{3,2}" : Outport
      mask Display: e = 0.06;c1 = [120 230 180]/255;c2 = ([120 230 180]+0)/(256+128);c3 = ([120 230 180]+128)/(256+128);patch([0 1 1 0],[0 0 1 1],c1);patch([0 1 1 1-e 1-e 0+e],[0 0 1 1-e 0+e 0+e],c2);patch([0 0 1 1-e 0+e 0+e],[0 1 1 1-e 1-e 0+e],c3);plot([0 1 1 0 0],[0 0 1 1 0]);
  wires:
  "p{3}"/1 -> mux/1
  mux/1 -> "pd{3,2}"/1

== system MLP_networks/net_col_e_f_4_5/Layer 3/LW{3,2} ==
  "ad{3,2}" : Inport  PortDimensions=40
      mask Display: e = 0.06;c1 = [120 230 180]/255;c2 = ([120 230 180]+0)/(256+128);c3 = ([120 230 180]+128)/(256+128);patch([0 1 1 0],[0 0 1 1],c1);patch([0 1 1 1-e 1-e 0+e],[0 0 1 1-e 0+e 0+e],c2);patch([0 0 1 1-e 0+e 0+e],[0 1 1 1-e 1-e 0+e],c3);plot([0 1 1 0 0],[0 0 1 1 0]);
  "IW{3,2}(1,:)'" : Constant  Value=[-0.96420633365073039;-0.56470894868679311;-0.026568931423403459;-0.62286137814214104;0.79975505344964437;-0.0047251761658306315;-1.1753588908027983;0.79703648674276117;-0.26077390194839112;-0.14762812450402174;0.20372858370056476;0.78220446346900241;0.42403446511291415;0.25214715040023983;-0.7697572703757295;0.20249608766121105;0.088323928113259217;0.56910310743673254;-0.95035012609665115;0.13483887108301593;0.52871744588626168;-0.95130436410373043;-0.36020596402288602;-0.096290781861516073;0.37984011617865188;-0.75203309716004263;0.89153436290847554;-0.65878513134658767;-0.29504614135789586;-0.30614325594878444;-0.40619861016866343;0.31676946466516936;0.57345688033427189;-0.55010621027475237;-0.18659234007791545;0.80054144734864829;-1.1811331396467935;0.94049514845871829;-0.89490932141341473;0.40666469974584835]
      mask Display: e = 0.06;c1 = [120 150 230]/255;c2 = ([120 150 230]+0)/383;c3 = ([120 150 230]+128)/383;patch([0 1 1 0],[0 0 1 1],c1);patch([0 1 1 1-e 1-e 0+e],[0 0 1 1-e 0+e 0+e],c2);patch([0 0 1 1-e 0+e 0+e],[0 1 1 1-e 1-e 0+e],c3);plot([0 1 1 0 0],[0 0 1 1 0]);disp('weights');
  Mux : Mux  Inputs=1
      mask Display: e = 0.06;c1 = [120 150 230]/255;c2 = ([120 150 230]+0)/383;c3 = ([120 150 230]+128)/383;patch([0 1 1 0],[0 0 1 1],c1);patch([0 1 1 1-e 1-e 0+e],[0 0 1 1-e 0+e 0+e],c2);patch([0 0 1 1-e 0+e 0+e],[0 1 1 1-e 1-e 0+e],c3);plot([0 1 1 0 0],[0 0 1 1 0]);disp('Mux');
  dotprod1 : neural/Weight Functions/dotprod  SystemSampleTime=-1
  "lz{3,2}" : Outport
      mask Display: e = 0.06;c1 = [120 230 180]/255;c2 = ([120 230 180]+0)/(256+128);c3 = ([120 230 180]+128)/(256+128);patch([0 1 1 0],[0 0 1 1],c1);patch([0 1 1 1-e 1-e 0+e],[0 0 1 1-e 0+e 0+e],c2);patch([0 0 1 1-e 0+e 0+e],[0 1 1 1-e 1-e 0+e],c3);plot([0 1 1 0 0],[0 0 1 1 0]);
  wires:
  "IW{3,2}(1,:)'"/1 -> dotprod1/1
  "ad{3,2}"/1 -> dotprod1/2
  dotprod1/1 -> Mux/1
  Mux/1 -> "lz{3,2}"/1

== system MLP_networks/net_col_e_f_5_6/Layer 1/Delays 1 ==
  "p{1}" : Inport  PortDimensions=2
      mask Display: e = 0.06;c1 = [120 230 180]/255;c2 = ([120 230 180]+0)/(256+128);c3 = ([120 230 180]+128)/(256+128);patch([0 1 1 0],[0 0 1 1],c1);patch([0 1 1 1-e 1-e 0+e],[0 0 1 1-e 0+e 0+e],c2);patch([0 0 1 1-e 0+e 0+e],[0 1 1 1-e 1-e 0+e],c3);plot([0 1 1 0 0],[0 0 1 1 0]);
  mux : Mux  Inputs=1
      mask Display: e = 0.06;c1 = [120 150 230]/255;c2 = ([120 150 230]+0)/383;c3 = ([120 150 230]+128)/383;patch([0 1 1 0],[0 0 1 1],c1);patch([0 1 1 1-e 1-e 0+e],[0 0 1 1-e 0+e 0+e],c2);patch([0 0 1 1-e 0+e 0+e],[0 1 1 1-e 1-e 0+e],c3);plot([0 1 1 0 0],[0 0 1 1 0]);disp('Mux')
  "pd{1,1}" : Outport
      mask Display: e = 0.06;c1 = [120 230 180]/255;c2 = ([120 230 180]+0)/(256+128);c3 = ([120 230 180]+128)/(256+128);patch([0 1 1 0],[0 0 1 1],c1);patch([0 1 1 1-e 1-e 0+e],[0 0 1 1-e 0+e 0+e],c2);patch([0 0 1 1-e 0+e 0+e],[0 1 1 1-e 1-e 0+e],c3);plot([0 1 1 0 0],[0 0 1 1 0]);
  wires:
  "p{1}"/1 -> mux/1
  mux/1 -> "pd{1,1}"/1
